simulink model "example_CollectorUnglazedinSubsystem"  (R2018b)
settings: Solver=ode45  StartTime=0.0  StopTime=24*3600  MaxStep=1800  RelTol=1e-3  EnableMultiTasking=on
undefined symbols (not defined in the file): collectorfilename, path_carnot
libraries: carnot x10
settings Model: DataDictionary=example_collectorUnglazedSLDD.sldd  Creator=drhf  LastModifiedBy=P41573
settings DataIOCC: LimitDataPoints=on  SaveFormat=Array
settings OptimizationCC: ExpressionDepthLimit=2147483647  LifeSpan=inf
settings DebuggingCC: UnderspecifiedInitializationDetection=Classic  MergeDetectMultiDrivingBlocksExec=none  SolverPrmCheckMsg=warning  StateNameClashWarn=warning  SFUnexpectedBacktrackingDiag=warning  SFNoUnconditionalDefaultTransitionDiag=warning  SFExecutionAtInitializationDiag=none
settings HardwareCC: ProdBitPerPointer=32  ProdBitPerSizeT=32  ProdBitPerPtrDiffT=32  ProdLargestAtomicFloat=None  ProdIntDivRoundTo=Undefined  ProdEndianess=Unspecified  ProdWordSize=32  ProdHWDeviceType=32-bit Generic
settings ModelReferenceCC: PropagateSignalLabelsOutOfModel=off
settings SFSimCC: SimUseLocalCustomCode=off
settings RTWCC: RTWUseLocalCustomCode=off
settings CodeAppCC: StateflowObjectComments=on
settings GRTTargetCC: TargetLangStandard=C89/C90 (ANSI)  GeneratePreprocessorConditionals=Disable all  CombineOutputUpdateFcns=off  GRTInterface=on
settings ConfigComp: CovMetricSettings=dw  CovHtmlReporting=on  CovSaveCumulativeToWorkspaceVar=on  CovSaveSingleToWorkspaceVar=on  CovExternalEMLEnable=off

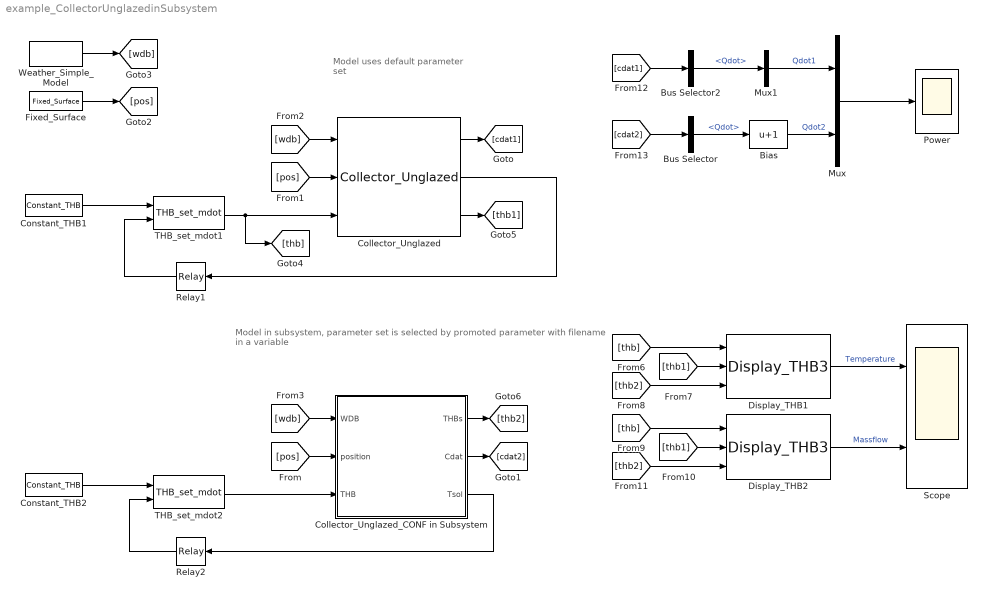
== system example_CollectorUnglazedinSubsystem ==
  note: Model uses default
      | parameter set
  note: Model in subsystem, parameter set is selected
      | by promoted parameter with filename in a variable
  Bias : Bias  Bias=1
  Bus Selector : BusSelector  OutputSignals=Qdot
  Bus Selector2 : BusSelector  OutputSignals=Qdot
  Collector_Unglazed : carnot/Source/Solar_Thermal/Collector_Unglazed  tini=22  Ncollector=1  PathName=fullfile(path_carnot('libsl'), 'Source', 'Solar_Thermal', 'Collector_Unglazed', 'parameter_set')  FileName='DefaultCollectorUnglazed.mat'  userPath=off  userParam=off  acol=2.5  len=2  nodes=10  fta=0.9  eps=0.9  u0l=40  u0c=1  u0g=40  u1l=8  u1c=1  u1g=8  u1e=0.01  hi=200  capa=5000  capf=4000  SensorTimeConstant=10  dplin=5504.4  dpqua=6222.096
      settings: SourceProductName=Carnot
  Collector_Unglazed_CONF in Subsystem : Subsystem  mask{PathName=fullfile(path_carnot('libsl'), 'Source', 'Solar_Thermal', 'Collector_Unglazed', 'parameter_set'), FileName=collectorfilename}
      mask prompts: PathName "Path"; FileName "Parameter set"
      mask TypeOptions PathName: Collector_Unglazed_CONF2/PathName
      mask TypeOptions FileName: Collector_Unglazed_CONF2/FileName
  Constant_THB1 : carnot/Source/Simple/Constant_THB  t=40  mdot=100/3600  p=1e5  mID=No Pressure Drop  fluid=Water  mix=0  mix2=0  mix3=0  dia=0.02  hgt=0
      settings: SourceProductName=Carnot
  Constant_THB2 : carnot/Source/Simple/Constant_THB  t=40  mdot=100/3600  p=1e5  mID=No Pressure Drop  fluid=Water  mix=0  mix2=0  mix3=0  dia=0.02  hgt=0
      settings: SourceProductName=Carnot
  Display_THB1 : carnot/Outputs/Display_THB3  t=on  m=off  p=off  id=off  mix=off  d=off
      settings: SourceProductName=Carnot
  Display_THB2 : carnot/Outputs/Display_THB3  t=off  m=on  p=off  id=off  mix=off  d=off
      settings: SourceProductName=Carnot
  Fixed_Surface : carnot/Weather/Fixed_Surface  colangle=30  colazi=0  colrot=0
      settings: SourceProductName=Carnot
  Mux : Mux  Inputs=2
  Mux1 : Mux  Inputs=1
  Power : Scope
  Relay1 : Relay  OnSwitchValue=47  OffSwitchValue=42  OnOutputValue=50/3600
  Relay2 : Relay  OnSwitchValue=47  OffSwitchValue=42  OnOutputValue=50/3600
  Scope : Scope  NumInputPorts=2
  THB_set_mdot1 : carnot/Source/Simple/THB_set_mdot
      settings: SourceProductName=Carnot
  THB_set_mdot2 : carnot/Source/Simple/THB_set_mdot
      settings: SourceProductName=Carnot
  Weather_Simple_Model : carnot/Weather/Weather_Simple_Model  Ibn=900  Idg=100  tamb=5  deltaTsky=-6  rh=50  precip="10e-3/24/3600           % 10 mm in 24 h"  cloud=0.125  p=1013e2  vw=1  wdir=270  lat=60  colangle=0  colazi=0  colrot=0
      settings: SourceProductName=Carnot
  wires:
  THB_set_mdot1/1 -> [thb], Collector_Unglazed/3
  Constant_THB1/1 -> THB_set_mdot1/1
  Collector_Unglazed/2 -> Relay1/1
  Relay1/1 -> THB_set_mdot1/2
  Relay2/1 -> THB_set_mdot2/2
  THB_set_mdot2/1 -> Collector_Unglazed_CONF in Subsystem/3(THB)
  Collector_Unglazed_CONF in Subsystem/3(Tsol) -> Relay2/1
  Display_THB1/1 -> Scope/1  "Temperature"
  Bus Selector/1 -> Bias/1  "<Qdot>"
  Mux/1 -> Power/1
  Display_THB2/1 -> Scope/2  "Massflow"
  Bias/1 -> Mux/2  "Qdot2"
  Bus Selector2/1 -> Mux1/1  "<Qdot>"
  [thb] -> Display_THB1/1
  [thb1] -> Display_THB1/2
  [thb2] -> Display_THB1/3
  [thb] -> Display_THB2/1
  [thb1] -> Display_THB2/2
  [thb2] -> Display_THB2/3
  Mux1/1 -> Mux/1  "Qdot1"
  [cdat1] -> Bus Selector2/1
  [cdat2] -> Bus Selector/1
  Collector_Unglazed/1 -> [cdat1]
  Collector_Unglazed_CONF in Subsystem/2(Cdat) -> [cdat2]
  Weather_Simple_Model/1 -> [wdb]
  Fixed_Surface/1 -> [pos]
  [pos] -> Collector_Unglazed_CONF in Subsystem/2(position)
  [pos] -> Collector_Unglazed/2
  [wdb] -> Collector_Unglazed/1
  [wdb] -> Collector_Unglazed_CONF in Subsystem/1(WDB)
  Constant_THB2/1 -> THB_set_mdot2/1
  Collector_Unglazed/3 -> [thb1]
  Collector_Unglazed_CONF in Subsystem/1(THBs) -> [thb2]

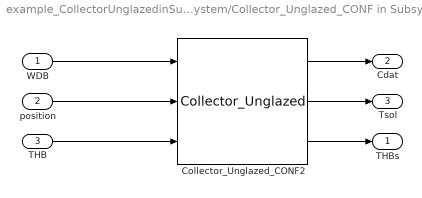
== system example_CollectorUnglazedinSubsystem/Collector_Unglazed_CONF in Subsystem ==
  WDB : Inport
  position : Inport  Port=2
  THB : Inport  Port=3
  Collector_Unglazed_CONF2 : carnot/Source/Solar_Thermal/Collector_Unglazed  tini=22  Ncollector=1  PathName=PathName  FileName=FileName  userPath=off  userParam=off  acol=2.5  len=2  nodes=10  fta=0.9  eps=0.9  u0l=40  u0c=1  u0g=40  u1l=8  u1c=1  u1g=8  u1e=0.01  hi=200  capa=5000  capf=4000  SensorTimeConstant=10  dplin=5504.4  dpqua=6222.096
      settings: SourceProductName=Carnot
  THBs : Outport
  Cdat : Outport  Port=2
  Tsol : Outport  Port=3
  wires:
  Collector_Unglazed_CONF2/1 -> Cdat/1
  THB/1 -> Collector_Unglazed_CONF2/3
  Collector_Unglazed_CONF2/2 -> Tsol/1
  Collector_Unglazed_CONF2/3 -> THBs/1
  position/1 -> Collector_Unglazed_CONF2/2
  WDB/1 -> Collector_Unglazed_CONF2/1
